simulink model "bicycle_complex"  (Simulink 8.8)
settings: Solver=ode45  StartTime=0.0  StopTime=10  MaxStep=1  RelTol=1e-3
settings Model: SuppressorTable=22 serialization::archive 11 0 3 0 0 0 11 0  Creator=root  LastModifiedBy=root
settings DataIOCC: LimitDataPoints=off  SaveFormat=Dataset  SignalLoggingSaveFormat=Dataset
settings DebuggingCC: UnderspecifiedInitializationDetection=Simplified  MergeDetectMultiDrivingBlocksExec=error  FcnCallInpInsideContextMsg=error  StateNameClashWarn=none  SFUnexpectedBacktrackingDiag=error  SFNoUnconditionalDefaultTransitionDiag=error
settings HardwareCC: ProdBitPerPointer=64  ProdBitPerSizeT=64  ProdBitPerPtrDiffT=64  ProdLargestAtomicFloat=Float  ProdIntDivRoundTo=Zero  ProdEndianess=LittleEndian  ProdWordSize=64  ProdHWDeviceType=Intel->x86-64 (Windows64)
settings ModelReferenceCC: PropagateSignalLabelsOutOfModel=on
settings GRTTargetCC: TargetLangStandard=C99 (ISO)  GeneratePreprocessorConditionals=Use local settings  CombineOutputUpdateFcns=on  GRTInterface=off
settings ConfigComp: CovMetricSettings=dwe  CovHtmlReporting=off  CovSaveCumulativeToWorkspaceVar=off  CovSaveSingleToWorkspaceVar=off  CovExternalEMLEnable=on

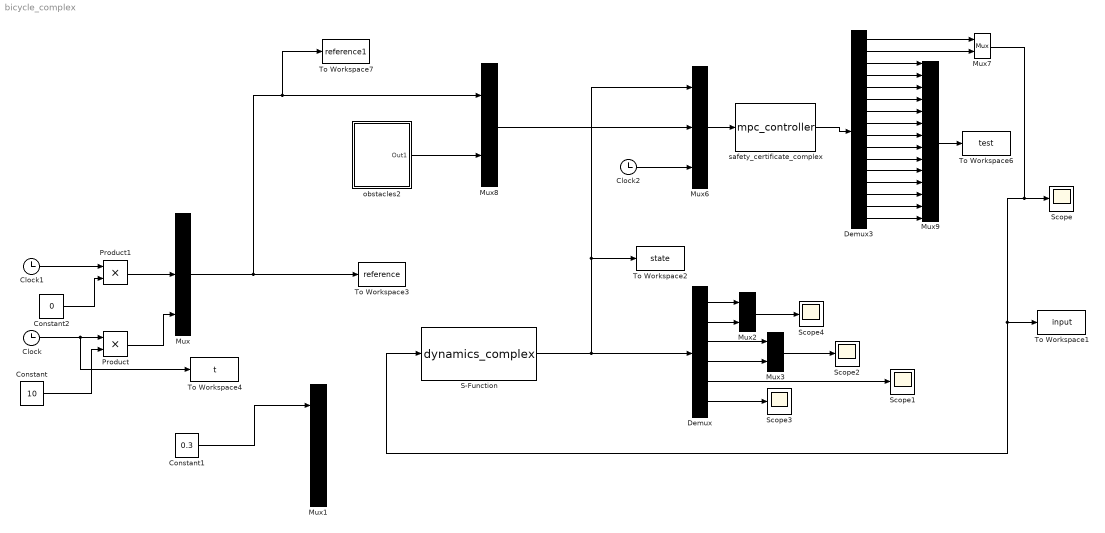
== system bicycle_complex ==
  Clock : Clock
  Clock1 : Clock
  Clock2 : Clock
  Constant : Constant  Value=10
  Constant1 : Constant  Value=0.3
  Constant2 : Constant  Value=0
  Demux : Demux  Outputs=6
  Demux3 : Demux  Outputs=16
  Mux : Mux  Inputs=3
  Mux1 : Mux  Inputs=3
  Mux{2..3,7..8} (4 alike) : Mux  Inputs=2
  Mux6 : Mux  Inputs=3
  Mux9 : Mux  Inputs=14
  Product : Product
  Product1 : Product
  S-Function : S-Function  FunctionName=dynamics_complex  SFunctionDeploymentMode=off  EnableBusSupport=off
  Scope{,1..4} (5 alike) : Scope
  To Workspace1 : ToWorkspace  VariableName=input  SampleTime=-1
  To Workspace2 : ToWorkspace  VariableName=state  SampleTime=-1
  To Workspace3 : ToWorkspace  VariableName=reference  SampleTime=-1
  To Workspace4 : ToWorkspace  VariableName=t  SampleTime=-1
  To Workspace6 : ToWorkspace  VariableName=test  SampleTime=-1
  To Workspace7 : ToWorkspace  VariableName=reference1  SampleTime=-1
  obstacles2 : Subsystem
  safety_certificate_complex : MATLABFcn  MATLABFcn=mpc_controller  OutputDimensions=16
  wires:
  Mux/1 -> To Workspace7/1, Mux8/1, To Workspace3/1
  S-Function/1 -> Demux/1, To Workspace2/1, Mux6/1
  Demux/1 -> Mux2/1
  Demux/2 -> Mux2/2
  Demux/3 -> Mux3/1
  Demux/4 -> Mux3/2
  Mux2/1 -> Scope4/1
  Mux3/1 -> Scope2/1
  Clock/1 -> To Workspace4/1, Product/1
  Constant/1 -> Product/2
  Constant2/1 -> Product1/2
  Clock1/1 -> Product1/1
  Mux6/1 -> safety_certificate_complex/1
  safety_certificate_complex/1 -> Demux3/1
  Demux3/1 -> Mux7/1
  Demux3/2 -> Mux7/2
  Mux7/1 -> Scope/1, To Workspace1/1, S-Function/1
  obstacles2/1(Out1) -> Mux8/2
  Mux9/1 -> To Workspace6/1
  Clock2/1 -> Mux6/3
  Product/1 -> Mux/3
  Product1/1 -> Mux/2
  Constant1/1 -> Mux1/1
  Demux/5 -> Scope1/1
  Demux/6 -> Scope3/1
  Mux8/1 -> Mux6/2
  Demux3/3 -> Mux9/1
  Demux3/4 -> Mux9/2
  Demux3/5 -> Mux9/3
  Demux3/6 -> Mux9/4
  Demux3/7 -> Mux9/5
  Demux3/8 -> Mux9/6
  Demux3/9 -> Mux9/7
  Demux3/10 -> Mux9/8
  Demux3/11 -> Mux9/9
  Demux3/12 -> Mux9/10
  Demux3/15 -> Mux9/13
  Demux3/14 -> Mux9/12
  Demux3/13 -> Mux9/11
  Demux3/16 -> Mux9/14

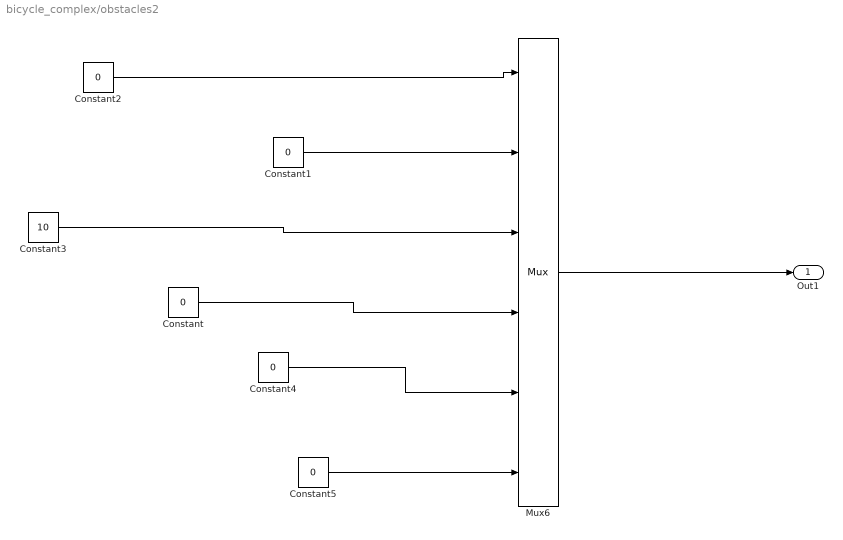
== system bicycle_complex/obstacles2 ==
  Constant{,1..2,4..5} (5 alike) : Constant  Value=0
  Constant3 : Constant  Value=10
  Mux6 : Mux  Inputs=6
  Out1 : Outport
  wires:
  Constant3/1 -> Mux6/3
  Constant1/1 -> Mux6/2
  Constant/1 -> Mux6/4
  Constant2/1 -> Mux6/1
  Mux6/1 -> Out1/1
  Constant4/1 -> Mux6/5
  Constant5/1 -> Mux6/6
